simulink model "lab11sm"  (R2021a)
settings: Solver=VariableStepAuto  StartTime=0.0  StopTime=10.0  RelTol=1e-3  AbsTol=1e-3  EnableMultiTasking=on
undefined symbols (not defined in the file): b1, b2, b3, F_1, F_2, F_3, time_F_1, time_F_2, time_F_3, x1_0, x2_0, x3_0
libraries: fl_lib x25, nesl_utility x16
settings Model: Creator=Alex  LastModifiedBy=Alex
settings SolverCC: AutoScaleAbsTol=off  AlgebraicLoopSolver=TrustRegion
settings DataIOCC: LimitDataPoints=on  MaxDataPoints=10000
settings OptimizationCC: LifeSpan=inf
settings DebuggingCC: AllowSymbolicDim=off  SFUnexpectedBacktrackingDiag=warning  SFNoUnconditionalDefaultTransitionDiag=warning  SFExecutionAtInitializationDiag=none  SFMachineParentedDataDiag=warning  ArithmeticOperatorsInVariantConditions=warning
settings SFSimCC: SimUseLocalCustomCode=off  CustomCodeUndefinedFunction=UseInterfaceOnly
settings RTWCC: RTWUseLocalCustomCode=off
settings CodeAppCC: StateflowObjectComments=on
settings GRTTargetCC: TargetLangStandard=C89/C90 (ANSI)
settings ConfigComp: CovMetricSettings=dw  CovSaveCumulativeToWorkspaceVar=on  CovSaveSingleToWorkspaceVar=on  CovExternalEMLEnable=off  CovSFcnEnable=off
settings SimscapeCC: SimscapeLogType=all  SimscapeLogSimulationStatistics=on  SimscapeLogDataHistory=10000

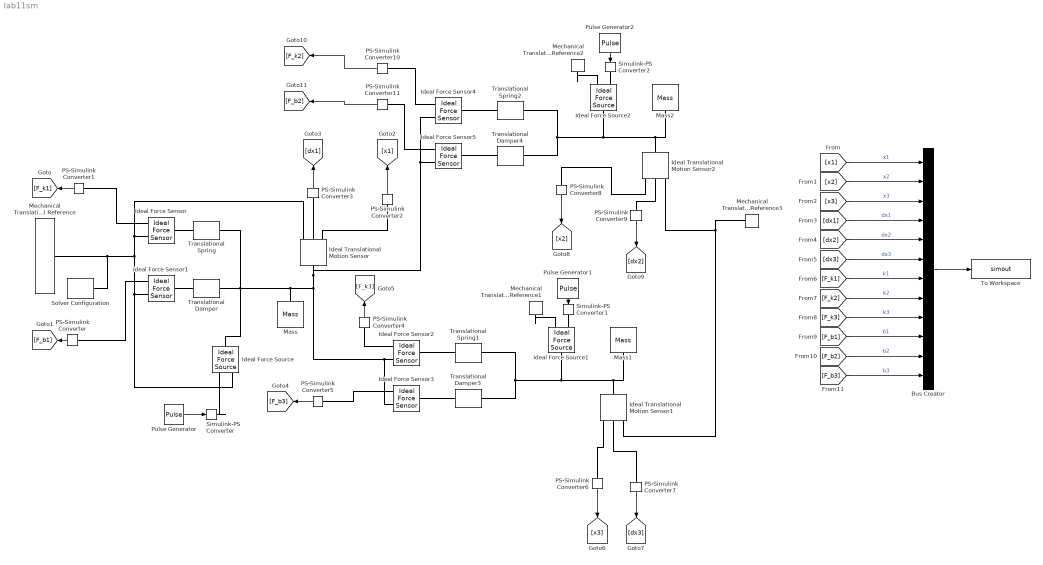
== system lab11sm ==
  Bus Creator : BusCreator  Inputs=12
  Ideal Force Sensor{,1..5} (6 alike) : fl_lib/Mechanical/Mechanical Sensors/Ideal Force Sensor
  Ideal Force Source : fl_lib/Mechanical/Mechanical Sources/Ideal Force Source
  Ideal Force Source1 : fl_lib/Mechanical/Mechanical Sources/Ideal Force Source
  Ideal Force Source2 : fl_lib/Mechanical/Mechanical Sources/Ideal Force Source
  Ideal Translational Motion Sensor : fl_lib/Mechanical/Mechanical Sensors/Ideal Translational Motion Sensor  offset=x1_0 m
  Ideal Translational Motion Sensor1 : fl_lib/Mechanical/Mechanical Sensors/Ideal Translational Motion Sensor  offset=x3_0 m
  Ideal Translational Motion Sensor2 : fl_lib/Mechanical/Mechanical Sensors/Ideal Translational Motion Sensor  offset=x2_0 m
  Mass : fl_lib/Mechanical/Translational Elements/Mass  mass=m1 kg  num_ports=foundation.enum.numPorts2.one  v_specify=off  v_priority=High  v=0 m/s  v_nominal_specify=off  v_nominal_unit=m/s  v_nominal_value=1  f_specify=off  f_priority=None  f=0 N  f_nominal_specify=off  f_nominal_unit=N  f_nominal_value=1
  Mass1 : fl_lib/Mechanical/Translational Elements/Mass  mass=m3 kg  num_ports=foundation.enum.numPorts2.one  v_specify=off  v_priority=High  v=0 m/s  v_nominal_specify=off  v_nominal_unit=m/s  v_nominal_value=1  f_specify=off  f_priority=None  f=0 N  f_nominal_specify=off  f_nominal_unit=N  f_nominal_value=1
  Mass2 : fl_lib/Mechanical/Translational Elements/Mass  mass=m2 kg  num_ports=foundation.enum.numPorts2.one  v_specify=off  v_priority=High  v=0 m/s  v_nominal_specify=off  v_nominal_unit=m/s  v_nominal_value=1  f_specify=off  f_priority=None  f=0 N  f_nominal_specify=off  f_nominal_unit=N  f_nominal_value=1
  Mechanical Translational Reference{,1..3} (4 alike) : fl_lib/Mechanical/Translational Elements/Mechanical Translational Reference
  PS-Simulink Converter{,1..11} (12 alike) : nesl_utility/PS-Simulink Converter  PhysicalDomain=network_engine_domain  SubClassName=ps_output  LeftPortType=input  RightPortType=output  PseudoPeriodic=off  Frequencies=[]  Unit=inherit  AffineConversion=off
      settings: SourceProductBaseCode=PW,SS
  Pulse Generator : DiscretePulseGenerator  PulseType=Time based  Amplitude=F_1  Period=t  PulseWidth=100 * time_F_1 / t
  Pulse Generator1 : DiscretePulseGenerator  PulseType=Time based  Amplitude=F_3  Period=t  PulseWidth=100 * time_F_3 / t
  Pulse Generator2 : DiscretePulseGenerator  PulseType=Time based  Amplitude=F_2  Period=t  PulseWidth="100 * time_F_2 /  t"
  Simulink-PS Converter : nesl_utility/Simulink-PS Converter  PhysicalDomain=network_engine_domain  SubClassName=ps_input  LeftPortType=input  RightPortType=output  PseudoPeriodic=off  Frequencies=[]  NoiseDistribution=none  NoiseParameters=[]  Unit=N  AffineConversion=off  FilteringAndDerivatives=provide  SimscapeFilterOrder=1  InputFilterTimeConstant=0.001  UdotUserProvided=0
      settings: SourceProductBaseCode=PW,SS
  Simulink-PS Converter1 : nesl_utility/Simulink-PS Converter  PhysicalDomain=network_engine_domain  SubClassName=ps_input  LeftPortType=input  RightPortType=output  PseudoPeriodic=off  Frequencies=[]  NoiseDistribution=none  NoiseParameters=[]  Unit=N  AffineConversion=off  FilteringAndDerivatives=provide  SimscapeFilterOrder=1  InputFilterTimeConstant=0.001  UdotUserProvided=0
      settings: SourceProductBaseCode=PW,SS
  Simulink-PS Converter2 : nesl_utility/Simulink-PS Converter  PhysicalDomain=network_engine_domain  SubClassName=ps_input  LeftPortType=input  RightPortType=output  PseudoPeriodic=off  Frequencies=[]  NoiseDistribution=none  NoiseParameters=[]  Unit=N  AffineConversion=off  FilteringAndDerivatives=provide  SimscapeFilterOrder=1  InputFilterTimeConstant=0.001  UdotUserProvided=0
      settings: SourceProductBaseCode=PW,SS
  Solver Configuration : nesl_utility/Solver Configuration  PhysicalDomain=network_engine_domain  SubClassName=solver  LeftPortType=input  RightPortType=generic  Tones=[]  Harmonics=[]  SimulateNoise=off  Profile=off  UseLocalSampling=off  EnableSwitchedLinearOptims=on  FrequencyDomain=off  UseCCode=off  RelTol=0.001  AbsTol=1e-06  MinStep=1e-09  ToWorkspace=off  RevertToSquareIcSolve=off  NumHomotopyIterations=100  PhasorMode=off  PhasorModeNumHarmonics=1  DoDC=off  ResidualTolerance=1e-09  UseLocalSolver=off  LocalSolverChoice=NE_BACKWARD_EULER_ADVANCER  LocalSolverSampleTime=0.001  DoFixedCost=off  MaxNonlinIter=3  MaxModeIter=2  ComputeImpulses=off  ImpulseIterations=2  LinearAlgebra=Sparse  EquationFormulation=NE_TIME_EF  DelaysMemoryBudget=1024  AutomaticFiltering=on  FilteringTimeConstant=0.001  PartitionStorageMethod=AS_NEEDED  PartitionMemoryBudget=1024  PartitionMethod=FAST
      settings: SourceProductBaseCode=PW,SS
  To Workspace : ToWorkspace  VariableName=simout  SaveFormat=Timeseries  SampleTime=-1
  Translational Damper : fl_lib/Mechanical/Translational Elements/Translational Damper  D=b1 N/(m/s)  v_specify=off  v_priority=None  v=0 m/s  v_nominal_specify=off  v_nominal_unit=m/s  v_nominal_value=1  f_specify=off  f_priority=None  f=0 N  f_nominal_specify=off  f_nominal_unit=N  f_nominal_value=1
  Translational Damper3 : fl_lib/Mechanical/Translational Elements/Translational Damper  D=b3 N/(m/s)  v_specify=off  v_priority=None  v=0 m/s  v_nominal_specify=off  v_nominal_unit=m/s  v_nominal_value=1  f_specify=off  f_priority=None  f=0 N  f_nominal_specify=off  f_nominal_unit=N  f_nominal_value=1
  Translational Damper4 : fl_lib/Mechanical/Translational Elements/Translational Damper  D=b2 N/(m/s)  v_specify=off  v_priority=None  v=0 m/s  v_nominal_specify=off  v_nominal_unit=m/s  v_nominal_value=1  f_specify=off  f_priority=None  f=0 N  f_nominal_specify=off  f_nominal_unit=N  f_nominal_value=1
  Translational Spring : fl_lib/Mechanical/Translational Elements/Translational Spring  spr_rate=k1 N/m  v_specify=off  v_priority=None  v=0 m/s  v_nominal_specify=off  v_nominal_unit=m/s  v_nominal_value=1  f_specify=off  f_priority=None  f=0 N  f_nominal_specify=off  f_nominal_unit=N  f_nominal_value=1  x_specify=on  x_priority=High  x=x1_0 m  x_nominal_specify=off  x_nominal_unit=m  x_nominal_value=1
  Translational Spring1 : fl_lib/Mechanical/Translational Elements/Translational Spring  spr_rate=k3 N/m  v_specify=off  v_priority=None  v=0 m/s  v_nominal_specify=off  v_nominal_unit=m/s  v_nominal_value=1  f_specify=off  f_priority=None  f=0 N  f_nominal_specify=off  f_nominal_unit=N  f_nominal_value=1  x_specify=on  x_priority=High  x=x3_0 - x1_0 m  x_nominal_specify=off  x_nominal_unit=m  x_nominal_value=1
  Translational Spring2 : fl_lib/Mechanical/Translational Elements/Translational Spring  spr_rate=k2 N/m  v_specify=off  v_priority=None  v=0 m/s  v_nominal_specify=off  v_nominal_unit=m/s  v_nominal_value=1  f_specify=off  f_priority=None  f=0 N  f_nominal_specify=off  f_nominal_unit=N  f_nominal_value=1  x_specify=on  x_priority=High  x=x2_0 - x1_0 m  x_nominal_specify=off  x_nominal_unit=m  x_nominal_value=1
  wires:
  Pulse Generator/1 -> Simulink-PS Converter/1
  PS-Simulink Converter1/1 -> [F_k1]
  PS-Simulink Converter/1 -> [F_b1]
  PS-Simulink Converter2/1 -> [x1]
  PS-Simulink Converter3/1 -> [dx1]
  Pulse Generator1/1 -> Simulink-PS Converter1/1
  PS-Simulink Converter5/1 -> [F_b3]
  PS-Simulink Converter4/1 -> [F_k3]
  PS-Simulink Converter7/1 -> [dx3]
  PS-Simulink Converter6/1 -> [x3]
  Pulse Generator2/1 -> Simulink-PS Converter2/1
  PS-Simulink Converter9/1 -> [dx2]
  PS-Simulink Converter8/1 -> [x2]
  PS-Simulink Converter11/1 -> [F_b2]
  PS-Simulink Converter10/1 -> [F_k2]
  [x1] -> Bus Creator/1  "x1"
  [x2] -> Bus Creator/2  "x2"
  [x3] -> Bus Creator/3  "x3"
  [dx1] -> Bus Creator/4  "dx1"
  [dx2] -> Bus Creator/5  "dx2"
  [dx3] -> Bus Creator/6  "dx3"
  [F_k1] -> Bus Creator/7  "k1"
  [F_k2] -> Bus Creator/8  "k2"
  [F_k3] -> Bus Creator/9  "k3"
  [F_b1] -> Bus Creator/10  "b1"
  [F_b2] -> Bus Creator/11  "b2"
  [F_b3] -> Bus Creator/12  "b3"
  Bus Creator/1 -> To Workspace/1
  connections:
  Ideal Force Sensor/LConn1 -- Translational Spring/RConn1
  Translational Damper/RConn1 -- Ideal Force Sensor1/LConn1
  PS-Simulink Converter/LConn1 -- Ideal Force Sensor1/RConn2
  Mechanical Translational Reference/LConn1 -- Solver Configuration/RConn1 -- Ideal Force Source/RConn2 -- Ideal Force Sensor1/RConn1 -- Ideal Translational Motion Sensor/RConn1 -- Ideal Force Sensor/RConn1
  PS-Simulink Converter1/LConn1 -- Ideal Force Sensor/RConn2
  Simulink-PS Converter/RConn1 -- Ideal Force Source/RConn1
  PS-Simulink Converter2/LConn1 -- Ideal Translational Motion Sensor/RConn3
  PS-Simulink Converter3/LConn1 -- Ideal Translational Motion Sensor/RConn2
  Ideal Force Sensor2/LConn1 -- Translational Spring1/RConn1
  Translational Damper3/RConn1 -- Ideal Force Sensor3/LConn1
  Simulink-PS Converter1/RConn1 -- Ideal Force Source1/RConn1
  Ideal Force Source/LConn1 -- Translational Damper/LConn1 -- Mass/LConn1 -- Ideal Force Sensor4/RConn1 -- Ideal Force Sensor5/RConn1 -- Ideal Translational Motion Sensor/LConn1 -- Ideal Force Sensor3/RConn1 -- Ideal Force Sensor2/RConn1 -- Translational Spring/LConn1
  Translational Spring1/LConn1 -- Translational Damper3/LConn1 -- Mass1/LConn1 -- Ideal Translational Motion Sensor1/LConn1 -- Ideal Force Source1/LConn1
  PS-Simulink Converter4/LConn1 -- Ideal Force Sensor2/RConn2
  PS-Simulink Converter5/LConn1 -- Ideal Force Sensor3/RConn2
  PS-Simulink Converter6/LConn1 -- Ideal Translational Motion Sensor1/RConn3
  PS-Simulink Converter7/LConn1 -- Ideal Translational Motion Sensor1/RConn2
  Ideal Force Source2/LConn1 -- Translational Damper4/LConn1 -- Translational Spring2/LConn1 -- Mass2/LConn1 -- Ideal Translational Motion Sensor2/LConn1
  Simulink-PS Converter2/RConn1 -- Ideal Force Source2/RConn1
  Translational Damper4/RConn1 -- Ideal Force Sensor5/LConn1
  PS-Simulink Converter9/LConn1 -- Ideal Translational Motion Sensor2/RConn2
  Ideal Force Sensor4/LConn1 -- Translational Spring2/RConn1
  PS-Simulink Converter8/LConn1 -- Ideal Translational Motion Sensor2/RConn3
  PS-Simulink Converter11/LConn1 -- Ideal Force Sensor5/RConn2
  PS-Simulink Converter10/LConn1 -- Ideal Force Sensor4/RConn2
  Mechanical Translational Reference1/LConn1 -- Ideal Force Source1/RConn2
  Mechanical Translational Reference2/LConn1 -- Ideal Force Source2/RConn2
  Ideal Translational Motion Sensor1/RConn1 -- Mechanical Translational Reference3/LConn1 -- Ideal Translational Motion Sensor2/RConn1
